simulink model "pendulum"  (R2023b)
settings: Solver=VariableStepAuto  StartTime=0.0  StopTime=10.0  MaxStep=0.01  RelTol=1e-3
undefined symbols (not defined in the file): I
libraries: simulink_extras x2
settings Model: Creator=maxaz  LastModifiedBy=maxaz

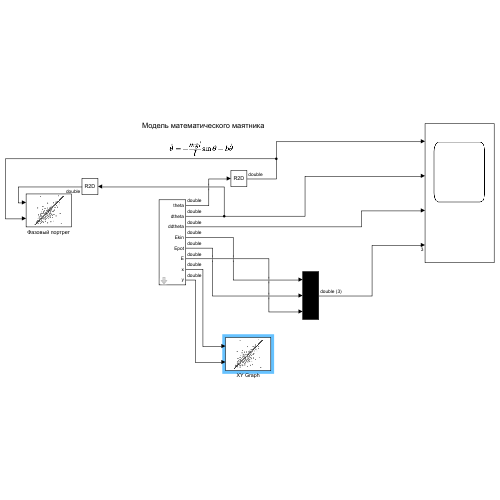
[thumbnail: Simulink's stored preview of the top-level diagram]
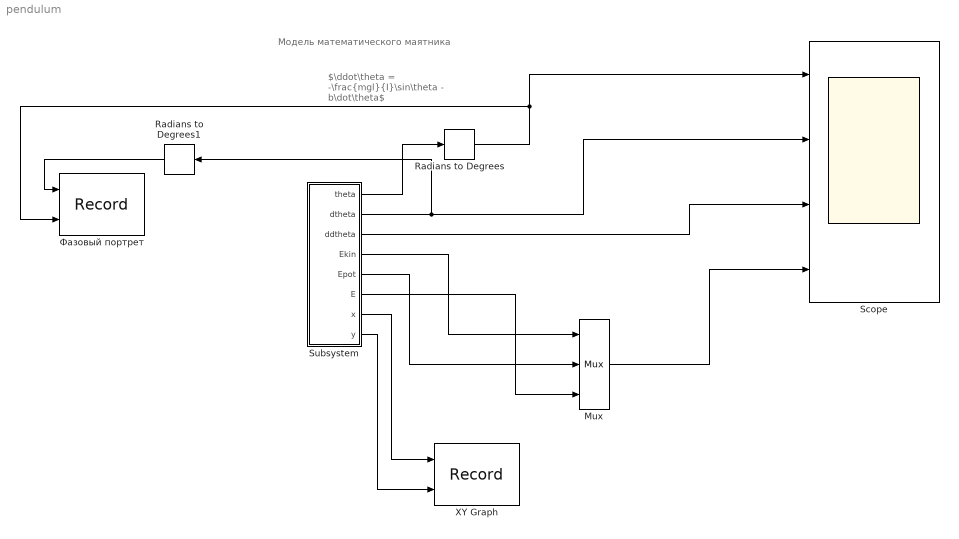
== system pendulum ==
  note: $\ddot\theta = -\frac{mgl}{I}\sin\theta - b\dot\theta$
  note: Модель математического маятника
  Mux : Mux  Inputs=3
  Radians to Degrees : simulink_extras/Transformations/Radians to Degrees
  Radians to Degrees1 : simulink_extras/Transformations/Radians to Degrees
  Scope : Scope  NumInputPorts=4
  Subsystem : Subsystem  mask{m=1, g=9.8, l=1, startDegree=30, b=0.3}
      mask prompts: m "Масса, кг"; g "Ускорение свободного падения, м/с^2"; l "Длина, м"; startDegree "Начальный угол, градусы"; b "Диссипативный коэффициент"
  XY Graph : Record  FileSettingsInternal="{\"entries\":[{\"content\":{\"excelSettings\":{\"content\":{},\"type\":\"Streamout.ExcelSettings\"}},\"type\":\"Streamout.FileSettingStorage\",\"uuid\":\"\"}],\"packageUris\":[\"http:\\/\\/schema.mathworks.com\\/mf0\\/streamout_blocks\\/R2020a\"],\"version\":\"1.0\"}"  Layout=[1 1]  SignalsInternal="{\"entries\":[{\"content\":{\"signals\":[{\"content\":{\"blockPath\":[],\"dimensions\":[1],\"domain\":\"\",\"lineColor\":\"#a2142f\",\"plots\":[1],\"port\":1,\"sid\":[\"\"],\"signalID\":398,\"signalName\":\"Subsystem:7\"},\"type\":\"RecordBlkView.Signal\",\"uuid\":\"\"},{\"content\":{\"blockPath\":[],\"dimensions\":[1],\"domain\":\"\",\"lineColor\":\"#139fff\",\"plots\":[1],\"port\":2,\"sid\":[\"\"],\"signalID\":402,\"signalName\":\"Subsystem:8\"},\"type\":\"RecordBlkView.Signal\",\"uuid\":\"\"}]},\"type\":\"RecordBlkView.InputSignals\",\"uuid\":\"\"}],\"packageUris\":[\"http:\\/\\/schema.mathworks.com\\/mf0\\/streamout_blocks\\/R2020a\"],\"version\":\"1.0\"}"  VisualizationBindings="{\"xyplotplugin\":{\"info\":[{\"series\":[{\"bindingParametersList\":[{\"parameter\":\"X-Axis\",\"signalID\":398,\"signalName\":\"Subsystem:7\"},{\"parameter\":\"Y-Axis\",\"signalID\":402,\"signalName\":\"Subsystem:8\"}],\"seriesID\":13182}],\"subplotID\":1}]}}"  CompatibilityTag=XY
  Фазовый портрет : Record  FileSettingsInternal="{\"entries\":[{\"content\":{\"excelSettings\":{\"content\":{},\"type\":\"Streamout.ExcelSettings\"}},\"type\":\"Streamout.FileSettingStorage\",\"uuid\":\"\"}],\"packageUris\":[\"http:\\/\\/schema.mathworks.com\\/mf0\\/streamout_blocks\\/R2020a\"],\"version\":\"1.0\"}"  Layout=[1 1]  SignalsInternal="{\"entries\":[{\"content\":{\"signals\":[{\"content\":{\"blockPath\":[],\"dimensions\":[1],\"domain\":\"\",\"lineColor\":\"#a2142f\",\"plots\":[1],\"port\":1,\"sid\":[\"\"],\"signalID\":406,\"signalName\":\"Radians\\nto Degrees1\"},\"type\":\"RecordBlkView.Signal\",\"uuid\":\"\"},{\"content\":{\"blockPath\":[],\"dimensions\":[1],\"domain\":\"\",\"lineColor\":\"#139fff\",\"plots\":[1],\"port\":2,\"sid\":[\"\"],\"signalID\":410,\"signalName\":\"Radians\\nto Degrees\"},\"type\":\"RecordBlkView.Signal\",\"uuid\":\"\"}]},\"type\":\"RecordBlkView.InputSignals\",\"uuid\":\"\"}],\"packageUris\":[\"http:\\/\\/schema.mathworks.com\\/mf0\\/streamout_blocks\\/R2020a\"],\"version\":\"1.0\"}"  VisualizationBindings="{\"xyplotplugin\":{\"info\":[{\"series\":[{\"bindingParametersList\":[{\"parameter\":\"X-Axis\",\"signalID\":406,\"signalName\":\"Radians\\nto Degrees1\"},{\"parameter\":\"Y-Axis\",\"signalID\":410,\"signalName\":\"Radians\\nto Degrees\"}],\"seriesID\":22523}],\"subplotID\":1}]}}"  CompatibilityTag=XY
  wires:
  Radians to Degrees/1 -> Фазовый портрет/2, Scope/1
  Subsystem/1(theta) -> Radians to Degrees/1
  Subsystem/2(dtheta) -> Radians to Degrees1/1, Scope/2
  Subsystem/3(ddtheta) -> Scope/3
  Subsystem/7(x) -> XY Graph/1
  Subsystem/8(y) -> XY Graph/2
  Subsystem/4(Ekin) -> Mux/1
  Subsystem/5(Epot) -> Mux/2
  Subsystem/6(E) -> Mux/3
  Mux/1 -> Scope/4
  Radians to Degrees1/1 -> Фазовый портрет/1

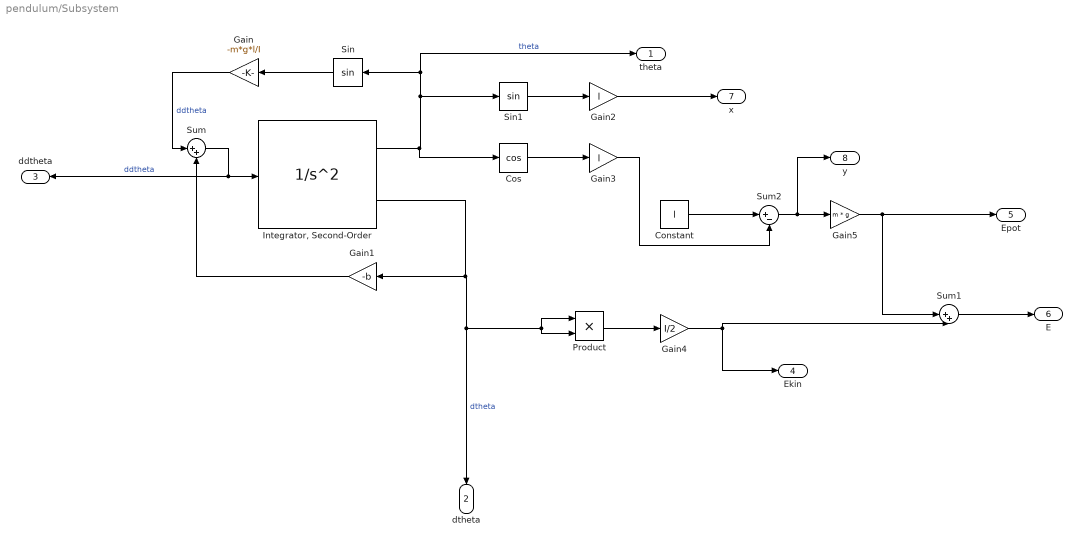
== system pendulum/Subsystem ==
  Constant : Constant  Value=l
  Cos : Trigonometry  Operator=cos
  Gain : Gain  Gain=-m*g*l/I
  Gain1 : Gain  Gain=-b
  Gain2 : Gain  Gain=l
  Gain3 : Gain  Gain=l
  Gain4 : Gain  Gain=I/2
  Gain5 : Gain  Gain=m * g
  "Integrator, Second-Order" : SecondOrderIntegrator  ICX=deg2rad(startDegree)
  Product : Product
  Sin : Trigonometry
  Sin1 : Trigonometry
  Sum : Sum  Inputs=|++
  Sum1 : Sum  Inputs=|++
  Sum2 : Sum  Inputs=|+-
  theta : Outport
  dtheta : Outport  Port=2
  ddtheta : Outport  Port=3
  Ekin : Outport  Port=4
  Epot : Outport  Port=5
  E : Outport  Port=6
  x : Outport  Port=7
  y : Outport  Port=8
  wires:
  "Integrator, Second-Order"/1 -> Cos/1, theta/1, Sin/1, Sin1/1  "theta"
  Sin/1 -> Gain/1
  Sum/1 -> "Integrator, Second-Order"/1, ddtheta/1  "ddtheta"
  "Integrator, Second-Order"/2 -> Product/2, Product/1, dtheta/1, Gain1/1  "dtheta"
  Gain1/1 -> Sum/2
  Gain/1 -> Sum/1  "ddtheta"
  Cos/1 -> Gain3/1
  Gain2/1 -> x/1
  Sin1/1 -> Gain2/1
  Gain3/1 -> Sum2/2
  Product/1 -> Gain4/1
  Gain5/1 -> Sum1/1, Epot/1
  Gain4/1 -> Sum1/2, Ekin/1
  Sum1/1 -> E/1
  Constant/1 -> Sum2/1
  Sum2/1 -> y/1, Gain5/1
